simulink model "ds_fivezone_cyberattack"  (R2020a)
settings: Solver=ode3  StartTime=182*24*3600  StopTime=183*24*3600  FixedStep=0.000001  RelTol=1e-3
undefined symbols (not defined in the file or in its folder): faultinjection__dy975f7hquM
settings Model: Creator=yangyang.fu  LastModifiedBy=yangyang.fu

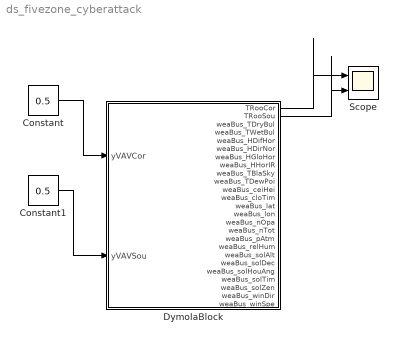
== system ds_fivezone_cyberattack ==
  Constant : Constant  Value=0.5  SampleTime=0.01
  Constant1 : Constant  Value=0.5  SampleTime=0.01
  DymolaBlock : Subsystem  Tag=07-Sep-2021 15:30:30#975  LoadFcn=if exist('newDymolaGui') newDymolaGui('ds_fivezone_cyberattack/DymolaBlock','PostLoadNew'); else error('Dymola not installed. Must install at least the file newDymolaGui.p'); end;
      mask help:
      | Dymola block.
      | A dymola block allows acausal physical modeling.
      | See Dymola manual for usage.
      settings: CopyFcn=newDymolaGui('07-Sep-2021 15:30:30#975','Copy');  DeleteFcn=if exist('newDymolaGui') newDymolaGui('ds_fivezone_cyberattack/DymolaBlock','Delete'); end;  NameChangeFcn=newDymolaGui('07-Sep-2021 15:30:30#975','Copy');  OpenFcn=newDymolaGui('ds_fivezone_cyberattack/DymolaBlock','Init');
      mask Display: image(reshape([1;1;1;1;1;1;1;1;1;1;1;1;1;1;1;1;1;1;1;1;1;1;0;0;0;0;0;0;0;0;0;0;1;1;1;1;1;1;1;1;0;1;1;1;1;1;1;1;1;0;1;1;1;1;1;0;0;0;0;0;0;0;1;1;0;0;0;0;0;0;0;1;1;0;0;0;0;0;0;0;1;1;0;0;0;0;0;0;0;1;1;0;0;0;0;0;0;0;1;1;0;0;0;0;0;0;0;1;1;0;0;0;0;0;0;0;1;1;0;0;0;0;0;0;0;1;1;0;0;0;0;0;0;0;1;1;0;0;0;0;0;0;0;1;1;0;0;0;0;0;0;0;1;1;0;0;0;0;0;0;0;1;1;0;0;0;0;0;0;0;1;1;0;0;0;0;0;0;0;1;1;0;0;0;0;0;0;0;1;1;0;0;0;0;0;0;0;1;1;0;0;0;0;0;0;0;1;1;0;0;0;0;0;0;0;1;1;0;0;0;0;0;0;0;1;1;0;0;0;0;0;0;0;1;1;0;0;0;0;0;0;0;1;1;0;0;0;0;0;0;0;1;1;0;0;0;0;0;0;0;1;1;0;0;0;0;0;0;0;1;1;1;1;1;0;1;1;1;1;1;1;1;1;0;1;1;1;1;1;1;1;1;0;0;0;0;0;0;0;0;0;0;1;1;1;1;1;1;1;1;1;1;1;1;1;1;1;1;1;1;1;1;1;1;1;1;1;1;1;1;1;1;1;1;1;1;1;1;1;1;1;1;1;1;1;1;0;0;0;0;0;0;0;0;0;0;1;1;1;1;1;1;1;1;0;1;1;1;1;1;1;1;1;0;1;1;1;1;1;0;0;0;0;0;0;0;1;1;0;0;0;0;0;0;0;1;1;0;0;0;0;0;0;0;1;1;0;0;0;0;0;0;0;1;1;0;0;0;0;0;0;0;1;1;0;0;0;0;0;0;0;1;1;0;0;0;0;0;0;0;1;1;0;0;0;0;0;0;0;1;1;0;0;0;0;0;0;0;1;1;0;0;0;0;0;0;0;1;1;0;0;0;0;0;0;0;1;1;0;0;0;0;0;0;0;1;1;0;0;0;0;0;0;0;1;1;0;0;0;0;0;0;0;1;1;0;0;0;0;0;0;0;1;1;0;0;0;0;0;0;0;1;1;0;0;0;0;0;0;0;1;1;0;0;0;0;0;0;0;1;1;0;0;0;0;0;0;0;1;1;0;0;0;0;0;0;0;1;1;0;0;0;0;0;0;0;1;1;0;0;0;0;0;0;0;1;1;0;0;0;0;0;0;0;1;1;0;0;0;0;0;0;0;1;1;1;1;1;0;1;1;1;1;1;1;1;1;0;1;1;1;1;1;1;1;1;0;0;0;0;0;0;0;0;0;0;1;1;1;1;1;1;1;1;1;1;1;1;1;1;1;1;1;1;1;1;1;1;1;1;1;1;1;1;1;1;1;1;1;1;1;1;1;1;1;1;1;1;1;1;0;0;0;0;0;0;0;0;0;0;1;1;1;1;1;1;1;1;0;1;1;1;1;1;1;1;1;0;1;1;1;1;1;0;0;0;0;0;0;0;1;1;0;0;0;0;0;0;0;1;1;0;1;1;1;1;1;0;1;1;0;1;1;1;1;1;0;1;1;0;1;1;1;1;1;0;1;1;0;1;1;1;1;1;0;1;1;0;1;1;1;1;1;0;1;1;0;1;1;1;1;1;0;1;1;0;1;1;1;1;1;0;1;1;0;1;1;1;1;1;0;1;1;0;1;1;1;1;1;0;1;1;0;1;1;1;1;1;0;1;1;0;1;1;1;1;1;0;1;1;0;1;1;1;1;1;0;1;1;0;1;1;1;1;1;0;1;1;0;1;1;1;1;1;0;1;1;0;1;1;1;1;1;0;1;1;0;1;1;1;1;1;0;1;1;0;1;1;1;1;1;0;1;1;0;1;1;1;1;1;0;1;1;0;1;1;1;1;1;0;1;1;0;1;1;1;1;1;0;1;1;0;0;0;0;0;0;0;1;1;0;0;0;0;0;0;0;1;1;1;1;1;0;1;1;1;1;1;1;1;1;0;1;1;1;1;1;1;1;1;0;0;0;0;0;0;0;0;0;0;1;1;1;1;1;1;1;1;1;1;1;1;1;1;1;1;1;1;1;1;1;1],18,18,3),[.2,.2,.6,.6])
  Scope : Scope  NumInputPorts=2
  wires:
  Constant/1 -> DymolaBlock/1(yVAVCor)
  Constant1/1 -> DymolaBlock/2(yVAVSou)
  DymolaBlock/1(TRooCor) -> Scope/1
  DymolaBlock/2(TRooSou) -> Scope/2

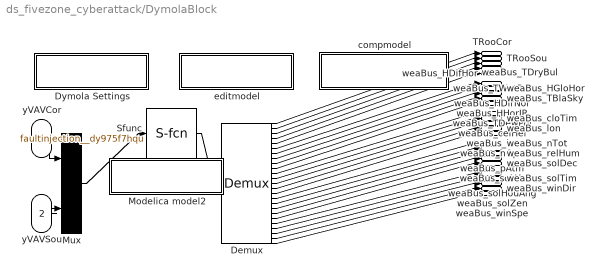
== system ds_fivezone_cyberattack/DymolaBlock ==
  yVAVCor : Inport
  yVAVSou : Inport  Port=2
  Demux : Demux  Outputs=[1;1;1;1;1;1;1;1;1;1;1;1;1;1;1;1;1;1;1;1;1;1;1;1;1]
  Dymola Settings : Subsystem  mask{ModelName=FaultInjection.HILSupport.BaselineSystem, MoFileName=D:/github/modelica-fault-library/FaultInjection/HILSupport/BaselineSystem.mo, dSpace=, BusConnector=[], ResultFile=[], ResultFileOnline=[], ResultDt=[], Libs=:, bigobj=[], ImportFolder=[], guimode=[], ModelName2=[], forRuntime=[], MEXLoad=[], omitDescription=[], ResultName=ds_cyber}
      mask prompts: ModelName "Name of Dymola model"; MoFileName "File Name (including .mo)"; ResultFile "Create Result"; ResultFileOnline "Load result"; ResultDt "Result min dt"; Libs "Used Libraries"; bigobj "Compiler flag /bigobj"; ImportFolder "Import folder"; guimode "GUI mode flag"; ModelName2 "Model name for import mode"; forRuntime "Runtime export"; MEXLoad "Compiled S-function"; omitDescription "Omit description strings"; ResultName "Name of result file"
      mask Display: disp('Dymola Settings');
  Modelica model2 : Subsystem
      mask Display: disp('Change parameters');
  Mux : Mux  Inputs=[1;1]
  Sfunc : S-Function  Tag=975f7hqu  FunctionName=faultinjection__dy975f7hqu  Parameters=[faultinjection__dy975f7hquM.pV],[faultinjection__dy975f7hquM.x0V]  PortCounts=[1;1]  SFunctionDeploymentMode=off  EnableBusSupport=off
      mask Display: image(imread('Dymola.bmp'))
  compmodel : Subsystem
      settings: OpenFcn=compileModelica('ds_fivezone_cyberattack/DymolaBlock');
      mask Display: disp('Compile Modelica model');
  editmodel : Subsystem
      settings: OpenFcn=editModelica('ds_fivezone_cyberattack/DymolaBlock');
      mask Display: disp('Edit Modelica model');
  TRooCor : Outport
  TRooSou : Outport  Port=2
  weaBus_TDryBul : Outport  Port=3
  weaBus_TWetBul : Outport  Port=4
  weaBus_HDifHor : Outport  Port=5
  weaBus_HDirNor : Outport  Port=6
  weaBus_HGloHor : Outport  Port=7
  weaBus_HHorIR : Outport  Port=8
  weaBus_TBlaSky : Outport  Port=9
  weaBus_TDewPoi : Outport  Port=10
  weaBus_ceiHei : Outport  Port=11
  weaBus_cloTim : Outport  Port=12
  weaBus_lat : Outport  Port=13
  weaBus_lon : Outport  Port=14
  weaBus_nOpa : Outport  Port=15
  weaBus_nTot : Outport  Port=16
  weaBus_pAtm : Outport  Port=17
  weaBus_relHum : Outport  Port=18
  weaBus_solAlt : Outport  Port=19
  weaBus_solDec : Outport  Port=20
  weaBus_solHouAng : Outport  Port=21
  weaBus_solTim : Outport  Port=22
  weaBus_solZen : Outport  Port=23
  weaBus_winDir : Outport  Port=24
  weaBus_winSpe : Outport  Port=25
  wires:
  Sfunc/1 -> Demux/1
  Demux/1 -> TRooCor/1
  Demux/2 -> TRooSou/1
  Demux/3 -> weaBus_TDryBul/1
  Demux/4 -> weaBus_TWetBul/1
  Demux/5 -> weaBus_HDifHor/1
  Demux/6 -> weaBus_HDirNor/1
  Demux/7 -> weaBus_HGloHor/1
  Demux/8 -> weaBus_HHorIR/1
  Demux/9 -> weaBus_TBlaSky/1
  Demux/10 -> weaBus_TDewPoi/1
  Demux/11 -> weaBus_ceiHei/1
  Demux/12 -> weaBus_cloTim/1
  Demux/13 -> weaBus_lat/1
  Demux/14 -> weaBus_lon/1
  Demux/15 -> weaBus_nOpa/1
  Demux/16 -> weaBus_nTot/1
  Demux/17 -> weaBus_pAtm/1
  Demux/18 -> weaBus_relHum/1
  Demux/19 -> weaBus_solAlt/1
  Demux/20 -> weaBus_solDec/1
  Demux/21 -> weaBus_solHouAng/1
  Demux/22 -> weaBus_solTim/1
  Demux/23 -> weaBus_solZen/1
  Demux/24 -> weaBus_winDir/1
  Demux/25 -> weaBus_winSpe/1
  Mux/1 -> Sfunc/1
  yVAVCor/1 -> Mux/1
  yVAVSou/1 -> Mux/2

== system ds_fivezone_cyberattack/DymolaBlock/Dymola Settings ==

== system ds_fivezone_cyberattack/DymolaBlock/Modelica model2 ==

== system ds_fivezone_cyberattack/DymolaBlock/compmodel ==

== system ds_fivezone_cyberattack/DymolaBlock/editmodel ==
